simulink subsystem "SOC_EKF_single_cell"  (R2024a)
settings: Solver=VariableStepAuto  StartTime=0.0  StopTime=10.0  RelTol=1e-3
values from neighbouring files (symbols this model uses):
  C1_charge = 9377.3935549443049 12784.352117101025 17780.50497472 16643.123985778271 9610.7814046871517 12434.390957717169 24208.147457962765 16643.123985778271 10958.451163474485 10412.733869794198 36077.185033058442 16284.188978791597 11087.989226120351 10412.721080978354 12558.892626131777 16284.132755832406 8400.05704109296 21527.466351599527 12559.044640816921 24292.09083057872 9668.09981772592 18067.5137    [CellDictionary.sldd]    (also in Gotion116CellDictionary.sldd)
  C1_discharge = 5874.2494091340313 5363.6664326091695 9522.8556893689238 9892.1424150937164 10573.648936441256 7509.1330056528359 12379.7123961796 11870.570898112459 14803.108511017757 9010.9596067834027 14855.654875415519 13057.627987923706 18124.826270932834 10256.216570725455 14394.082737985691 17344.683234031148 18123.650240143656 16753.837812941278 15223.664122901331 17105.94370428707 15393.257233666067 1709    [CellDictionary.sldd]    (also in Gotion116CellDictionary.sldd)
  C2_charge = 83286.762427651513 89132.1866794698 45094.898404433654 102834.93280571439 76741.821108505683 89132.1866794698 59590.039122816386 102834.93280571439 65813.629482078031 79325.3765455145 95053.590465977191 103252.50754873879 75221.9872077796 92085.153884857646 108235.64389779975 124119.58318976025 86474.809603960442 100146.15577427745 131936.69476387632 142532.08371487851 88887.819496347336 103155.57    [CellDictionary.sldd]    (also in Gotion116CellDictionary.sldd)
  C2_discharge = 8660.4321560409171 12676.055410309849 77918.08252980643 54468.490022335107 25981.29646812275 38028.16623092955 124668.93204769031 87149.584035736174 51962.5929362455 68450.6992156732 174536.50486676642 104579.50084288341 91872.675879310656 104895.79878604764 132964.7148052869 121894.93826354244 108633.64026784211 125213.15849032688 133235.68520284505 146107.42960041706 111988.29621948414 144386.68    [CellDictionary.sldd]    (also in Gotion116CellDictionary.sldd)
  C3_charge = 977235.776567173 1071975.4393548302 1300351.5011858649 2191683.7691258113 984479.59299833479 1033998.6902691127 1249089.2201867439 3148515.1881727232 996831.91383817617 1238576.5710734406 1713169.73062763 4327347.5647436548 1527057.3820877771 2924502.33319176 5986934.6241272911 5470254.34360569 1820703.5255430271 2277475.3277036194 5470247.2559996136 6319308.9695259091 2155412.4937486737 2698600.3    [CellDictionary.sldd]    (also in Gotion116CellDictionary.sldd)
  C3_discharge = 1055.9004514656031 12835.215816146119 947476.12402523274 507451.53207819723 10559.004514656031 64176.0790807306 1894952.2480504655 913412.7577407551 105590.04514656033 320880.395403653 2842428.3720756983 1278777.860837057 1002516.4759829378 1961294.7618454231 687275.55966035358 2345676.351051935 861318.16112133558 1416659.0872175139 2651384.6531096334 1308983.9983718023 796193.22889958438 1171144.    [CellDictionary.sldd]    (also in Gotion116CellDictionary.sldd)
  cell_capacity_nominal = 116.0    [CellDictionary.sldd]    (also in Gotion116CellDictionary.sldd)
  ECM_SOC : value not decoded    [CellDictionary.sldd]
  ECM_T : value not decoded    [CellDictionary.sldd]
  OCV_SOC : value not decoded    [CellDictionary.sldd]
  OCV_T : value not decoded    [CellDictionary.sldd]
  OCV_V = 3.089975 3.1958025155770748 3.2700856729308603 3.3269062967469782 3.3701558672655878 3.3935018471075473 3.4031249999999997 3.4106750000000003 3.417975 3.4255687342956502 3.4340073517474323 3.44463535689108 3.4571649659479133 3.4695529273207848 3.481325 3.49315 3.5048949462107366 3.5157966467267432 3.5254768755401917 3.534725 3.543897510782176 3.5528756373568848 3.5611426187731481 3.5686 3.575725 3    [CellDictionary.sldd]    (also in Gotion116CellDictionary.sldd; ParametersDataDictionary.sldd = 3.426 3.511 3.595 3.627 3.656 3.705 3.785 3.893 3.955 4.054 ; SOXDictionary.sldd = 3.426 3.511 3.595 3.627 3.656 3.705 3.785 3.893 3.955 4.054 ; SOXDictionaryGotion.sldd = 2.8 3.089975 3.1958025155770748 3.2700856729308603 3.3269062)
  R0_charge = 0.0011762548470330098 0.00082374580425955042 0.000528220046847626 0.00036375900896813311 0.0010441063780583621 0.00072163805067231468 0.00050986311152455624 0.00035574030260694049 0.0010321299216333078 0.00071105826266249655 0.00048266835826310457 0.00035372216488075841 0.001024720077996646 0.00069001121087368356 0.00048481817133183287 0.00034648647498852108 0.001011799939308299 0.0006697964359567    [CellDictionary.sldd]    (also in Gotion116CellDictionary.sldd)
  R0_discharge = 0.0011713156680267826 0.00080379131757867114 0.00053584971835591568 0.00037332457313021659 0.0011487629449379545 0.00077055056377129218 0.00052328698011887883 0.00035835507369999319 0.0011266444560462821 0.0007386844798434178 0.00050172364877783509 0.0003498356430994423 0.0010850138368129973 0.00069989297656780321 0.00047637432800705728 0.00034196489943770015 0.0010386918064711587 0.00065988337212    [CellDictionary.sldd]    (also in Gotion116CellDictionary.sldd)
  R1_charge = 0.00046991497657839924 0.0010779816764740048 0.00013720748025427109 0.00054498496863974164 0.00046376138253324481 0.00066376489201272156 0.00013720748025427109 0.00018528267520728436 0.00041621818829090906 0.00049349026745049 0.00020770204245624234 0.00018502550552971592 0.00041621893904479396 0.00049355079737852447 0.00036345316071937457 0.00018502550475278616 0.00030655167459223354 0.00020155261    [CellDictionary.sldd]    (also in Gotion116CellDictionary.sldd)
  R1_discharge = 0.00062343910396692745 0.00088344565476029683 0.000473998175802181 0.00030361323697364274 0.00034635505775940415 0.00063103261054306924 0.0003646139813862931 0.00025301103081136895 0.00024739646982814583 0.00052586050878589109 0.00030384498448857757 0.00023001002801033537 0.00022490588166195074 0.00047805500798717366 0.00027622271317143414 0.00021905716953365273 0.00022546269140634405 0.0003001510    [CellDictionary.sldd]    (also in Gotion116CellDictionary.sldd)
  R2_charge = 0.0013071970907491625 0.0011565350014947392 0.00094770363400168442 0.00027803074491849166 0.0011296066387324344 0.00079964133367552734 0.000585621349864987 0.00040094855176715479 0.00096825717163721565 0.00071275071905804873 0.00050086266287882315 0.00022186351951754667 0.000858047601085684 0.00068372107937354906 0.00048716119953890212 0.00021951334854306714 0.00082371775210131749 0.00056587719522    [CellDictionary.sldd]    (also in Gotion116CellDictionary.sldd)
  R2_discharge = 0.0082023616629522487 0.00477357645651923 0.0013535754139770782 0.00071689319983068869 0.0027341205543174162 0.0015911921521730766 0.00084598463373567378 0.00044805824989418042 0.0013670602771587081 0.00088399564009615365 0.00060427473838262416 0.00037338187491181703 0.00091137351810580548 0.00073666303341346137 0.00050356228198552015 0.0003556017856303019 0.00092980892733805819 0.0007515620058816    [CellDictionary.sldd]    (also in Gotion116CellDictionary.sldd)
  R3_charge = 0.0022791079484232404 0.00076358338365525792 0.0012549156736722906 0.00058631541275341111 0.0012276125164720909 0.00076358338365525792 0.00035824943217463234 0.00076079543468179163 0.0011171764499634 0.00069457337864931717 0.00035533139001579984 0.00094337886181821427 0.0006671085355807189 0.00046891528577433023 0.00033689307388307945 0.00072524071500878735 0.00058184070468519759 0.000371910545995    [CellDictionary.sldd]    (also in Gotion116CellDictionary.sldd)
  R3_discharge = 0.5961801788597515 0.049373498218042031 0.0017231068556688191 0.0031135501588106253 0.05961801788597515 0.0098746996436084068 0.00086155342783440954 0.0017297500882281251 0.0059618017885975146 0.0019749399287216814 0.00057436895188960632 0.0012355357773058038 0.000993633631432919 0.00065831330957389386 0.0004418222706843125 0.0011232143430052761 0.0013277019879200426 0.00096507261335108377 0.00043    [CellDictionary.sldd]    (also in Gotion116CellDictionary.sldd)
  soc_estim_init = 0.5    [EstimatorsDictionary.sldd]
  Ts = 1.0    [EstimatorsDictionary.sldd]    (also in batteryStateTransition.m = u(3))
libraries: sharedTrackingLibrary x1
settings Model: DataDictionary=EstimatorsDictionary.sldd  EnableAccessToBaseWorkspace=off  Creator=mmackenzie  LastModifiedBy=mmackenzie

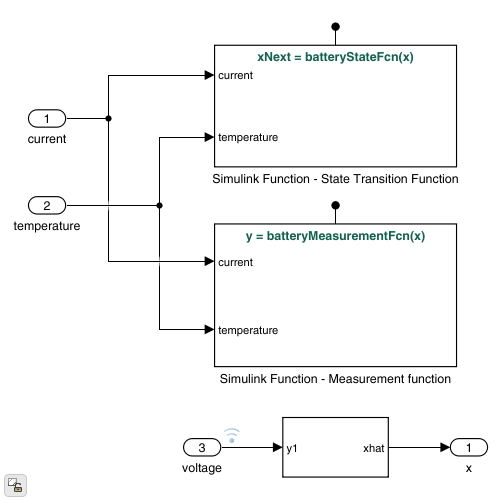
[thumbnail: Simulink's stored preview of the top-level diagram]
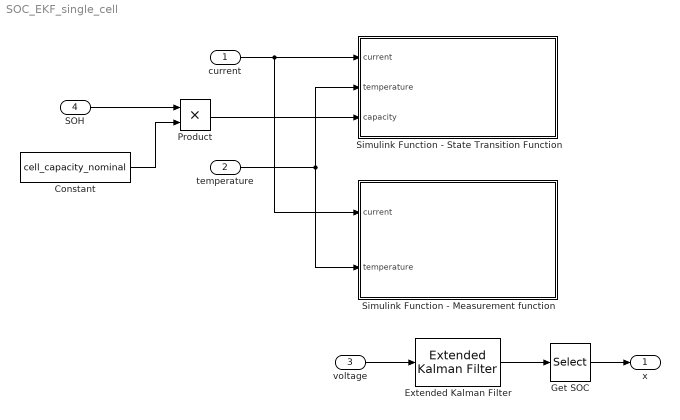
== system SOC_EKF_single_cell ==
  current : Inport
  temperature : Inport  Port=2
  voltage : Inport  Port=3
  SOH : Inport  Port=4
  Constant : Constant  Value=cell_capacity_nominal
  Extended Kalman Filter : sharedTrackingLibrary/Extended Kalman Filter  StateTransitionFcn=batteryStateFcn  HasStateTransitionJacobianFcn=off  HasAdditiveProcessNoise=Additive  ProcessNoise=state_covariance  HasTimeVaryingProcessNoise=off  HasStateTransitionFcnExtraArgument=0  InitialState=[soc_estim_init; 0; 0; 0]  InitialStateCovariance=initial_covariance  MeasurementFcn1=batteryMeasurementFcn  HasMeasurementJacobianFcn1=off  HasMeasurementEnablePort1=off  HasAdditiveMeasurementNoise1=Additive  MeasurementNoise1=measurement_covariance  HasTimeVaryingMeasurementNoise1=off  HasMeasurementFcnExtraArgument1=0  HasMeasurementWrapping1=off  MeasurementFcn2=myMeasurementFcn  HasMeasurementJacobianFcn2=off  HasMeasurementEnablePort2=off  HasAdditiveMeasurementNoise2=Additive  MeasurementNoise2=1  HasTimeVaryingMeasurementNoise2=off  HasMeasurementFcnExtraArgument2=0  HasMeasurementWrapping2=off  MeasurementFcn3=myMeasurementFcn  HasMeasurementJacobianFcn3=off  HasMeasurementEnablePort3=off  HasAdditiveMeasurementNoise3=Additive  MeasurementNoise3=1  HasTimeVaryingMeasurementNoise3=off  HasMeasurementFcnExtraArgument3=0  HasMeasurementWrapping3=off  MeasurementFcn4=myMeasurementFcn  HasMeasurementJacobianFcn4=off  HasMeasurementEnablePort4=off  HasAdditiveMeasurementNoise4=Additive  MeasurementNoise4=1  HasTimeVaryingMeasurementNoise4=off  HasMeasurementFcnExtraArgument4=0  HasMeasurementWrapping4=off  MeasurementFcn5=myMeasurementFcn  HasMeasurementJacobianFcn5=off  HasMeasurementEnablePort5=off  HasAdditiveMeasurementNoise5=Additive  MeasurementNoise5=1  HasTimeVaryingMeasurementNoise5=off  HasMeasurementFcnExtraArgument5=0  HasMeasurementWrapping5=off  EnableMultirate=off  StateTransitionFcnSampleTime=1  MeasurementFcn1SampleTime=1  MeasurementFcn2SampleTime=1  MeasurementFcn3SampleTime=1  MeasurementFcn4SampleTime=1  MeasurementFcn5SampleTime=1  UseCurrentEstimator=on  OutputStateCovariance=off  DataType=double  SampleTime=Ts  NumberOfMeasurements=1
      settings: LibrarySourceBlock=slident/Estimators/Extended Kalman Filter
  Get SOC : Selector  InputPortWidth=4  IndexOptions=Index vector (dialog)  Indices=1  OutputSizes=1
  Product : Product
  Simulink Function - Measurement function : Subsystem  TreatAsAtomicUnit=on
  Simulink Function - State Transition Function : Subsystem  TreatAsAtomicUnit=on
  x : Outport
  wires:
  temperature/1 -> Simulink Function - State Transition Function/2(temperature), Simulink Function - Measurement function/2(temperature)
  voltage/1 -> Extended Kalman Filter/1
  Extended Kalman Filter/1 -> Get SOC/1
  current/1 -> Simulink Function - State Transition Function/1(current), Simulink Function - Measurement function/1(current)
  Constant/1 -> Product/2
  SOH/1 -> Product/1
  Product/1 -> Simulink Function - State Transition Function/3(capacity)
  Get SOC/1 -> x/1

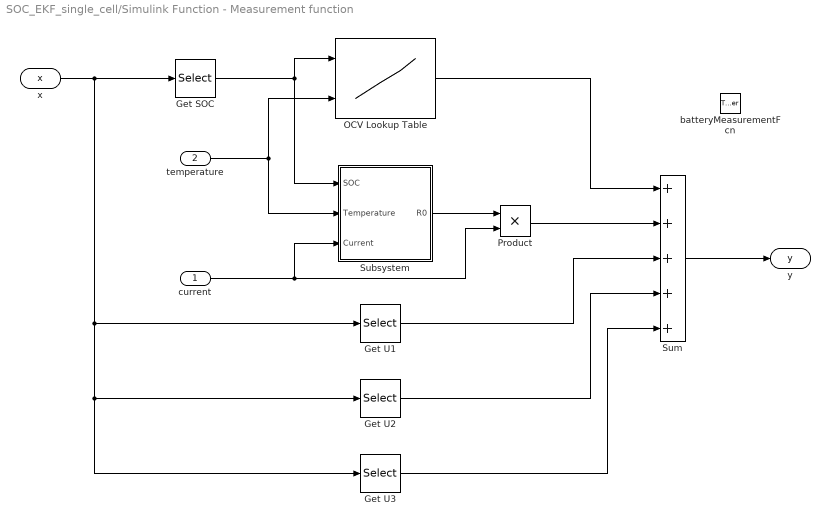
== system SOC_EKF_single_cell/Simulink Function - Measurement function ==
  current : Inport
  temperature : Inport  Port=2
  batteryMeasurementFcn : TriggerPort  TriggerType=function-call  IsSimulinkFunction=on  FunctionName=batteryMeasurementFcn  FunctionVisibility=scoped  VariantControl=(inherit)
  Get SOC : Selector  InputPortWidth=4  IndexOptions=Index vector (dialog)  Indices=1  OutputSizes=1
  Get U1 : Selector  InputPortWidth=4  IndexOptions=Index vector (dialog)  Indices=2  OutputSizes=1
  Get U2 : Selector  InputPortWidth=4  IndexOptions=Index vector (dialog)  Indices=3  OutputSizes=1
  Get U3 : Selector  InputPortWidth=4  IndexOptions=Index vector (dialog)  Indices=4  OutputSizes=1
  OCV Lookup Table : Lookup_n-D  BreakpointsForDimension1=OCV_SOC  BreakpointsForDimension2=OCV_T  Table=OCV_V  InternalRulePriority=Speed  RndMeth=Simplest
      settings: InputPortMap=u0,u1
  Product : Product
  Subsystem : Subsystem
  Sum : Sum  Inputs=+++++
  x : ArgIn  DisableCoverage=on  PortDimensions=4  ArgumentName=x
  y : ArgOut  DisableCoverage=on  ArgumentName=y
  wires:
  x/1 -> Get U3/1, Get U2/1, Get U1/1, Get SOC/1
  Get SOC/1 -> OCV Lookup Table/1, Subsystem/1(SOC)
  temperature/1 -> Subsystem/2(Temperature), OCV Lookup Table/2
  current/1 -> Product/2, Subsystem/3(Current)
  Subsystem/1(R0) -> Product/1
  OCV Lookup Table/1 -> Sum/1
  Product/1 -> Sum/2
  Get U1/1 -> Sum/3
  Get U2/1 -> Sum/4
  Get U3/1 -> Sum/5
  Sum/1 -> y/1

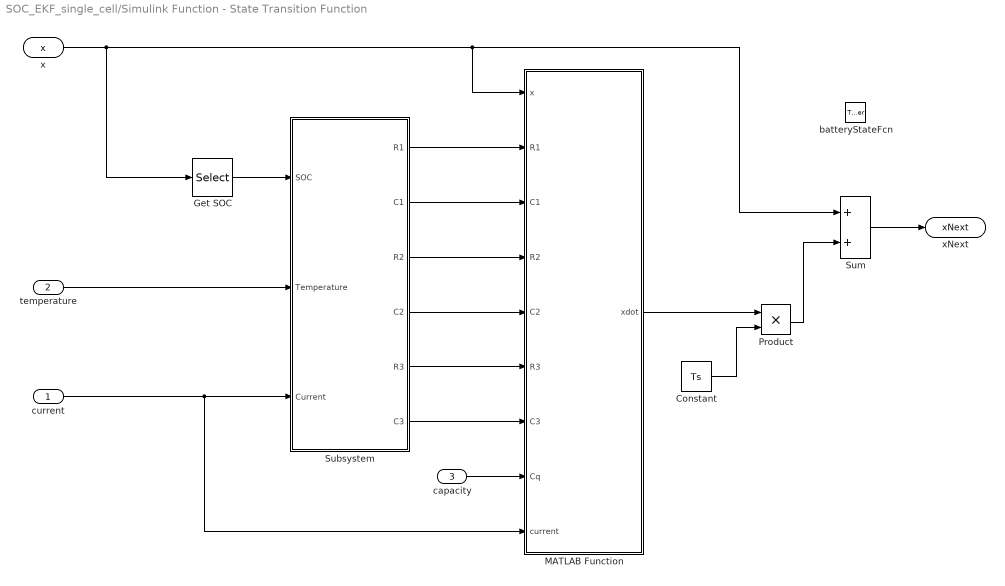
== system SOC_EKF_single_cell/Simulink Function - State Transition Function ==
  current : Inport
  temperature : Inport  Port=2
  capacity : Inport  Port=3
  batteryStateFcn : TriggerPort  TriggerType=function-call  IsSimulinkFunction=on  FunctionName=batteryStateFcn  FunctionVisibility=scoped  VariantControl=(inherit)
  Constant : Constant  Value=Ts
  Get SOC : Selector  InputPortWidth=4  IndexOptions=Index vector (dialog)  Indices=1  OutputSizes=1
  MATLAB Function : MATLAB Function  TreatAsAtomicUnit=on
  Product : Product
  Subsystem : Subsystem
  Sum : Sum
  x : ArgIn  DisableCoverage=on  PortDimensions=4  ArgumentName=x
  xNext : ArgOut  DisableCoverage=on  PortDimensions=4  ArgumentName=xNext
  wires:
  Subsystem/6(C3) -> MATLAB Function/7(C3)
  Subsystem/5(R3) -> MATLAB Function/6(R3)
  Subsystem/4(C2) -> MATLAB Function/5(C2)
  Subsystem/3(R2) -> MATLAB Function/4(R2)
  Subsystem/2(C1) -> MATLAB Function/3(C1)
  Subsystem/1(R1) -> MATLAB Function/2(R1)
  x/1 -> MATLAB Function/1(x), Sum/1, Get SOC/1
  Get SOC/1 -> Subsystem/1(SOC)
  temperature/1 -> Subsystem/2(Temperature)
  capacity/1 -> MATLAB Function/8(Cq)
  current/1 -> Subsystem/3(Current), MATLAB Function/9(current)
  Sum/1 -> xNext/1
  Constant/1 -> Product/2
  MATLAB Function/1(xdot) -> Product/1
  Product/1 -> Sum/2

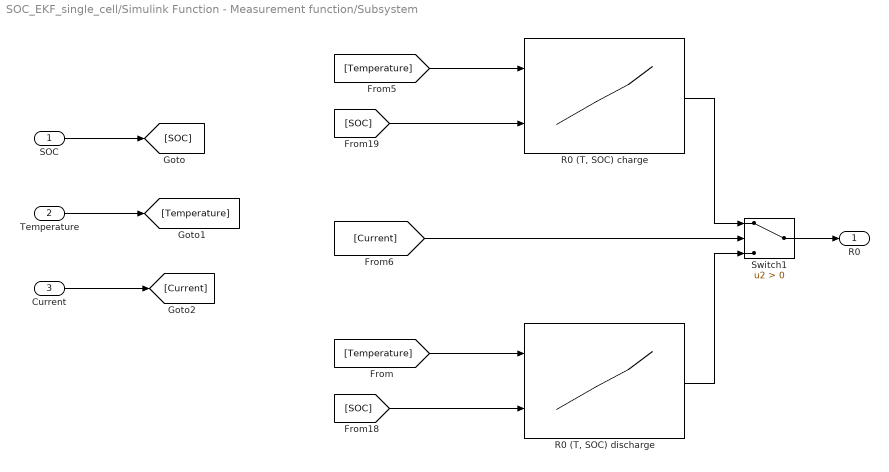
== system SOC_EKF_single_cell/Simulink Function - Measurement function/Subsystem ==
  SOC : Inport
  Temperature : Inport  Port=2
  Current : Inport  Port=3
  "R0 (T, SOC) charge" : Lookup_n-D  BreakpointsForDimension1=ECM_T  BreakpointsForDimension2=ECM_SOC  Table=R0_charge  InternalRulePriority=Speed  RndMeth=Simplest
      settings: InputPortMap=u0,u1
  "R0 (T, SOC) discharge" : Lookup_n-D  BreakpointsForDimension1=ECM_T  BreakpointsForDimension2=ECM_SOC  Table=R0_discharge  InternalRulePriority=Speed  RndMeth=Simplest
      settings: InputPortMap=u0,u1
  Switch1 : Switch  Criteria=u2 > Threshold  SaturateOnIntegerOverflow=off  InputSameDT=off
  R0 : Outport
  wires:
  "R0 (T, SOC) discharge"/1 -> Switch1/3
  "R0 (T, SOC) charge"/1 -> Switch1/1
  [SOC] -> "R0 (T, SOC) charge"/2
  [SOC] -> "R0 (T, SOC) discharge"/2
  [Temperature] -> "R0 (T, SOC) charge"/1
  [Temperature] -> "R0 (T, SOC) discharge"/1
  Current/1 -> [Current]
  Temperature/1 -> [Temperature]
  SOC/1 -> [SOC]
  Switch1/1 -> R0/1
  [Current] -> Switch1/2

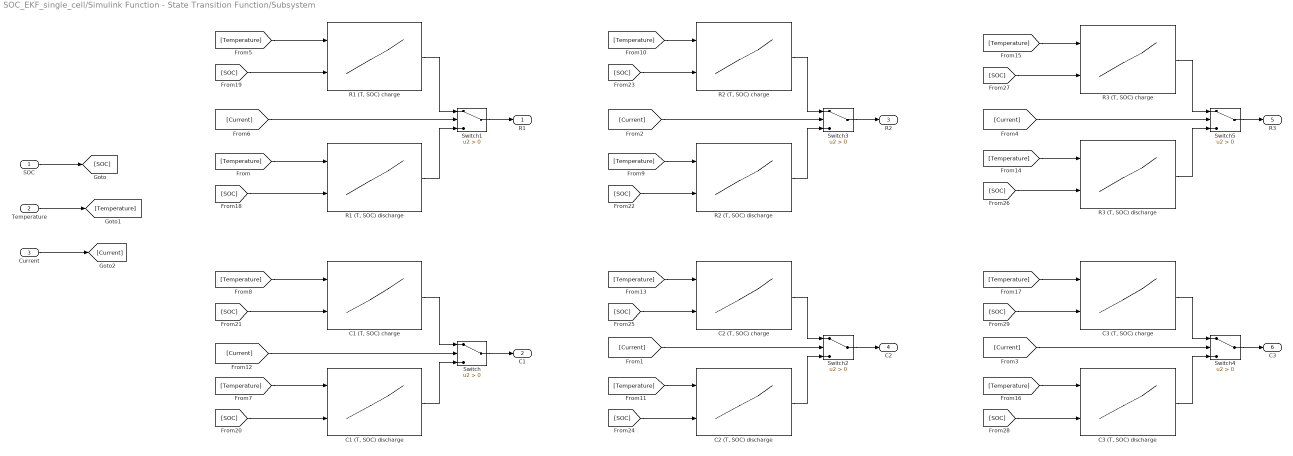
== system SOC_EKF_single_cell/Simulink Function - State Transition Function/Subsystem ==
  SOC : Inport
  Temperature : Inport  Port=2
  Current : Inport  Port=3
  "C1 (T, SOC) charge" : Lookup_n-D  BreakpointsForDimension1=ECM_T  BreakpointsForDimension2=ECM_SOC  Table=C1_charge  InternalRulePriority=Speed  RndMeth=Simplest
      settings: InputPortMap=u0,u1
  "C1 (T, SOC) discharge" : Lookup_n-D  BreakpointsForDimension1=ECM_T  BreakpointsForDimension2=ECM_SOC  Table=C1_discharge  InternalRulePriority=Speed  RndMeth=Simplest
      settings: InputPortMap=u0,u1
  "C2 (T, SOC) charge" : Lookup_n-D  BreakpointsForDimension1=ECM_T  BreakpointsForDimension2=ECM_SOC  Table=C2_charge  InternalRulePriority=Speed  RndMeth=Simplest
      settings: InputPortMap=u0,u1
  "C2 (T, SOC) discharge" : Lookup_n-D  BreakpointsForDimension1=ECM_T  BreakpointsForDimension2=ECM_SOC  Table=C2_discharge  InternalRulePriority=Speed  RndMeth=Simplest
      settings: InputPortMap=u0,u1
  "C3 (T, SOC) charge" : Lookup_n-D  BreakpointsForDimension1=ECM_T  BreakpointsForDimension2=ECM_SOC  Table=C3_charge  InternalRulePriority=Speed  RndMeth=Simplest
      settings: InputPortMap=u0,u1
  "C3 (T, SOC) discharge" : Lookup_n-D  BreakpointsForDimension1=ECM_T  BreakpointsForDimension2=ECM_SOC  Table=C3_discharge  InternalRulePriority=Speed  RndMeth=Simplest
      settings: InputPortMap=u0,u1
  "R1 (T, SOC) charge" : Lookup_n-D  BreakpointsForDimension1=ECM_T  BreakpointsForDimension2=ECM_SOC  Table=R1_charge  InternalRulePriority=Speed  RndMeth=Simplest
      settings: InputPortMap=u0,u1
  "R1 (T, SOC) discharge" : Lookup_n-D  BreakpointsForDimension1=ECM_T  BreakpointsForDimension2=ECM_SOC  Table=R1_discharge  InternalRulePriority=Speed  RndMeth=Simplest
      settings: InputPortMap=u0,u1
  "R2 (T, SOC) charge" : Lookup_n-D  BreakpointsForDimension1=ECM_T  BreakpointsForDimension2=ECM_SOC  Table=R2_charge  InternalRulePriority=Speed  RndMeth=Simplest
      settings: InputPortMap=u0,u1
  "R2 (T, SOC) discharge" : Lookup_n-D  BreakpointsForDimension1=ECM_T  BreakpointsForDimension2=ECM_SOC  Table=R2_discharge  InternalRulePriority=Speed  RndMeth=Simplest
      settings: InputPortMap=u0,u1
  "R3 (T, SOC) charge" : Lookup_n-D  BreakpointsForDimension1=ECM_T  BreakpointsForDimension2=ECM_SOC  Table=R3_charge  InternalRulePriority=Speed  RndMeth=Simplest
      settings: InputPortMap=u0,u1
  "R3 (T, SOC) discharge" : Lookup_n-D  BreakpointsForDimension1=ECM_T  BreakpointsForDimension2=ECM_SOC  Table=R3_discharge  InternalRulePriority=Speed  RndMeth=Simplest
      settings: InputPortMap=u0,u1
  Switch{,1..5} (6 alike) : Switch  Criteria=u2 > Threshold  SaturateOnIntegerOverflow=off  InputSameDT=off
  R1 : Outport
  C1 : Outport  Port=2
  R2 : Outport  Port=3
  C2 : Outport  Port=4
  R3 : Outport  Port=5
  C3 : Outport  Port=6
  wires:
  "C3 (T, SOC) discharge"/1 -> Switch4/3
  "C3 (T, SOC) charge"/1 -> Switch4/1
  "R3 (T, SOC) discharge"/1 -> Switch5/3
  "R3 (T, SOC) charge"/1 -> Switch5/1
  "C2 (T, SOC) charge"/1 -> Switch2/1
  "C2 (T, SOC) discharge"/1 -> Switch2/3
  "R2 (T, SOC) discharge"/1 -> Switch3/3
  "R2 (T, SOC) charge"/1 -> Switch3/1
  "C1 (T, SOC) discharge"/1 -> Switch/3
  "C1 (T, SOC) charge"/1 -> Switch/1
  "R1 (T, SOC) discharge"/1 -> Switch1/3
  "R1 (T, SOC) charge"/1 -> Switch1/1
  [SOC] -> "C3 (T, SOC) charge"/2
  [SOC] -> "C3 (T, SOC) discharge"/2
  [SOC] -> "R3 (T, SOC) charge"/2
  [SOC] -> "R3 (T, SOC) discharge"/2
  [SOC] -> "C2 (T, SOC) charge"/2
  [SOC] -> "C2 (T, SOC) discharge"/2
  [SOC] -> "R2 (T, SOC) charge"/2
  [SOC] -> "R2 (T, SOC) discharge"/2
  [SOC] -> "C1 (T, SOC) charge"/2
  [SOC] -> "C1 (T, SOC) discharge"/2
  [SOC] -> "R1 (T, SOC) charge"/2
  [SOC] -> "R1 (T, SOC) discharge"/2
  [Temperature] -> "C3 (T, SOC) charge"/1
  [Temperature] -> "C3 (T, SOC) discharge"/1
  [Temperature] -> "R3 (T, SOC) charge"/1
  [Temperature] -> "R3 (T, SOC) discharge"/1
  [Temperature] -> "C2 (T, SOC) charge"/1
  [Temperature] -> "C2 (T, SOC) discharge"/1
  [Temperature] -> "R2 (T, SOC) charge"/1
  [Temperature] -> "R2 (T, SOC) discharge"/1
  [Temperature] -> "C1 (T, SOC) charge"/1
  [Temperature] -> "C1 (T, SOC) discharge"/1
  [Temperature] -> "R1 (T, SOC) charge"/1
  [Temperature] -> "R1 (T, SOC) discharge"/1
  Current/1 -> [Current]
  Temperature/1 -> [Temperature]
  SOC/1 -> [SOC]
  Switch4/1 -> C3/1
  Switch1/1 -> R1/1
  Switch5/1 -> R3/1
  Switch3/1 -> R2/1
  Switch2/1 -> C2/1
  [Current] -> Switch2/2
  [Current] -> Switch5/2
  [Current] -> Switch/2
  Switch/1 -> C1/1
  [Current] -> Switch3/2
  [Current] -> Switch1/2
  [Current] -> Switch4/2

== matlab function SOC_EKF_single_cell/Simulink Function - State Transition Function/MATLAB Function ==
  data: x input; xdot output; R1 input; C1 input; R2 input; C2 input; R3 input; C3 input; Cq input; current input
function xdot = fcn(x, R1, C1, R2, C2, R3, C3, Cq, current)
xdot = zeros(size(x));
U1 = x(2);
U2 = x(3);
U3 = x(4);
xdot(1) = current / (3600 * Cq);
xdot(2) = -1 / (R1 * C1) * U1 + current / C1;
xdot(3) = -1 / (R2 * C2) * U2 + current / C2;
xdot(4) = -1 / (R3 * C3) * U3 + current / C3;
